simulink library "Quaternion"  (R2018b)
settings: Solver=VariableStepAuto  StartTime=0.0  StopTime=10.0  RelTol=1e-3
undefined symbols (not defined in the file): Newton, Raphson
libraries: $bdroot x8, AP_Math x3
settings Model: Creator=JCZou  LastModifiedBy=zouji
settings CodeAppCC: StateflowObjectComments=on

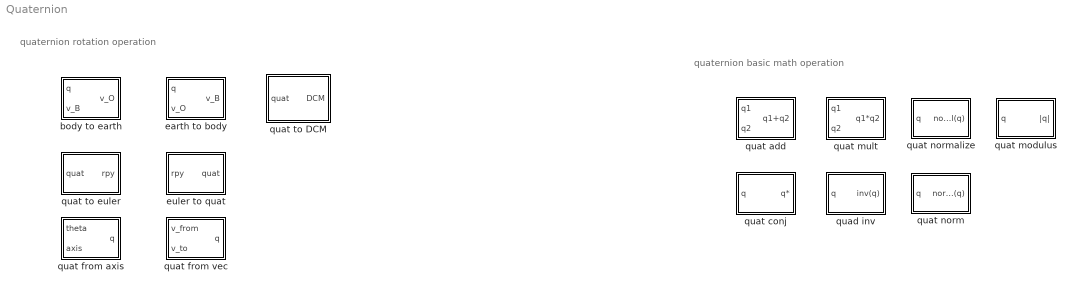
== system Quaternion ==
  note: quaternion rotation operation
  note: quaternion basic math operation
  body to earth : Subsystem
  earth to body : Subsystem
  euler to quat : Subsystem
  quad inv : Subsystem
  quat add : Subsystem
  quat conj : Subsystem
  quat from axis : Subsystem
  quat from vec : Subsystem
  quat modulus : Subsystem
  quat mult : Subsystem
  quat norm : Subsystem
  quat normalize : Subsystem
  quat to DCM : Subsystem
  quat to euler : Subsystem

== system Quaternion/body to earth ==
  q : Inport  Unit=1
  v_B : Inport  Port=2
  Mux : Mux  Inputs=3
  Subsystem : Subsystem
  Subsystem1 : Subsystem
  Subsystem2 : Subsystem
  quat normalize : $bdroot/quat normalize  SystemSampleTime=-1
  v_O : Outport
  wires:
  v_B/1 -> Subsystem/2(vec), Subsystem2/2(vec), Subsystem1/2(vec)
  quat normalize/1 -> Subsystem/1(q), Subsystem2/1(q), Subsystem1/1(q)
  Mux/1 -> v_O/1
  Subsystem1/1(V2) -> Mux/2
  Subsystem/1(V1) -> Mux/1
  Subsystem2/1(V3) -> Mux/3
  q/1 -> quat normalize/1

== system Quaternion/earth to body ==
  q : Inport  Unit=1
  v_O : Inport  Port=2
  Mux : Mux  Inputs=3
  Subsystem : Subsystem
  Subsystem1 : Subsystem
  Subsystem2 : Subsystem
  quat normalize : $bdroot/quat normalize  SystemSampleTime=-1
  v_B : Outport
  wires:
  v_O/1 -> Subsystem/2(vec), Subsystem2/2(vec), Subsystem1/2(vec)
  Subsystem1/1(V2) -> Mux/2
  Mux/1 -> v_B/1
  Subsystem/1(V1) -> Mux/1
  quat normalize/1 -> Subsystem2/1(q1), Subsystem1/1(q1), Subsystem/1(q1)
  q/1 -> quat normalize/1
  Subsystem2/1(V3) -> Mux/3

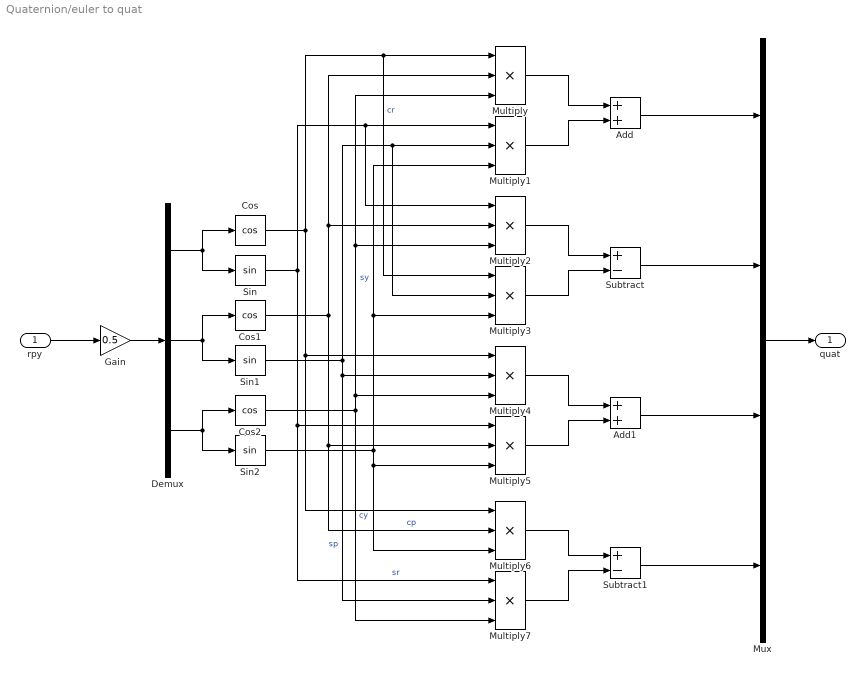
== system Quaternion/euler to quat ==
  rpy : Inport
  Add : Sum  OutDataTypeStr=Inherit: Same as first input
  Add1 : Sum  OutDataTypeStr=Inherit: Same as first input
  Cos : Trigonometry  Operator=cos
  Cos1 : Trigonometry  Operator=cos
  Cos2 : Trigonometry  Operator=cos
  Demux : Demux  Outputs=3
  Gain : Gain  Gain=0.5  OutDataTypeStr=Inherit: Same as input
  Multiply{,1..7} (8 alike) : Product  Inputs=3  OutDataTypeStr=Inherit: Same as first input
  Mux : Mux
  Sin : Trigonometry
  Sin1 : Trigonometry
  Sin2 : Trigonometry
  Subtract : Sum  Inputs=+-  OutDataTypeStr=Inherit: Same as first input
  Subtract1 : Sum  Inputs=+-  OutDataTypeStr=Inherit: Same as first input
  quat : Outport
  wires:
  rpy/1 -> Gain/1
  Gain/1 -> Demux/1
  Demux/1 -> Sin/1, Cos/1
  Demux/2 -> Cos1/1, Sin1/1
  Demux/3 -> Cos2/1, Sin2/1
  Cos/1 -> Multiply4/1, Multiply6/1, Multiply3/1, Multiply/1  "cr"
  Sin/1 -> Multiply5/1, Multiply7/1, Multiply2/1, Multiply1/1  "sr"
  Cos1/1 -> Multiply5/2, Multiply6/2, Multiply/2, Multiply2/2  "cp"
  Sin1/1 -> Multiply4/2, Multiply7/2, Multiply3/2, Multiply1/2  "sp"
  Cos2/1 -> Multiply7/3, Multiply4/3, Multiply/3, Multiply2/3  "cy"
  Sin2/1 -> Multiply5/3, Multiply6/3, Multiply1/3, Multiply3/3  "sy"
  Multiply/1 -> Add/1
  Multiply1/1 -> Add/2
  Multiply2/1 -> Subtract/1
  Multiply3/1 -> Subtract/2
  Multiply4/1 -> Add1/1
  Multiply5/1 -> Add1/2
  Multiply6/1 -> Subtract1/1
  Multiply7/1 -> Subtract1/2
  Mux/1 -> quat/1
  Add/1 -> Mux/1
  Subtract/1 -> Mux/2
  Add1/1 -> Mux/3
  Subtract1/1 -> Mux/4

== system Quaternion/quad inv ==
  q : Inport
  Divide : Product  Inputs=*/
  quat conj : $bdroot/quat conj  SystemSampleTime=-1
  quat norm : $bdroot/quat norm  SystemSampleTime=-1
  inv(q) : Outport
  wires:
  q/1 -> quat conj/1, quat norm/1
  quat conj/1 -> Divide/1
  quat norm/1 -> Divide/2
  Divide/1 -> inv(q)/1

== system Quaternion/quat add ==
  q1 : Inport
  q2 : Inport  Port=2
  Add : Sum  OutDataTypeStr=Inherit: Same as first input
  q1+q2 : Outport
  wires:
  Add/1 -> q1+q2/1
  q1/1 -> Add/1
  q2/1 -> Add/2

== system Quaternion/quat conj ==
  q : Inport
  Demux : Demux
  Gain : Gain  Gain=-1  OutDataTypeStr=Inherit: Same as input
  Gain1 : Gain  Gain=-1  OutDataTypeStr=Inherit: Same as input
  Gain2 : Gain  Gain=-1  OutDataTypeStr=Inherit: Same as input
  Mux : Mux
  q* : Outport
  wires:
  q/1 -> Demux/1
  Demux/2 -> Gain/1
  Demux/1 -> Mux/1
  Demux/3 -> Gain1/1
  Demux/4 -> Gain2/1
  Mux/1 -> q*/1
  Gain/1 -> Mux/2
  Gain1/1 -> Mux/3
  Gain2/1 -> Mux/4

== system Quaternion/quat from axis ==
  theta : Inport
  axis : Inport  Port=2
  Cos : Trigonometry  Operator=cos
  Demux : Demux  Outputs=3
  Gain : Gain  Gain=0.5  OutDataTypeStr=Inherit: Same as input
  Multiply : Product  OutDataTypeStr=Inherit: Same as first input
  Multiply1 : Product  OutDataTypeStr=Inherit: Same as first input
  Multiply2 : Product  OutDataTypeStr=Inherit: Same as first input
  Mux : Mux
  Sin : Trigonometry
  quat normalize : $bdroot/quat normalize  SystemSampleTime=-1
  q : Outport
  wires:
  theta/1 -> Gain/1
  Gain/1 -> Cos/1, Sin/1
  Mux/1 -> quat normalize/1
  Cos/1 -> Mux/1
  axis/1 -> Demux/1
  Sin/1 -> Multiply2/1, Multiply1/1, Multiply/1
  Demux/1 -> Multiply/2
  Multiply/1 -> Mux/2
  Multiply1/1 -> Mux/3
  Multiply2/1 -> Mux/4
  Demux/2 -> Multiply1/2
  Demux/3 -> Multiply2/2
  quat normalize/1 -> q/1

== system Quaternion/quat from vec ==
  v_from : Inport
  v_to : Inport  Port=2
  Acos : Trigonometry  Operator=acos
  Cos : Trigonometry  Operator=cos
  Demux : Demux  Outputs=3
  Dot Product : DotProduct  InputSameDT=on  OutDataTypeStr=Inherit: Inherit via internal rule
  Gain : Gain  Gain=0.5  OutDataTypeStr=Inherit: Same as input
  Multiply1 : Product
  Multiply2 : Product
  Multiply3 : Product
  Mux : Mux
  Sin : Trigonometry
  cross_product : AP_Math/cross_product  SystemSampleTime=-1
  quat normalize : $bdroot/quat normalize  SystemSampleTime=-1
  vec_normalize : AP_Math/vec_normalize  SystemSampleTime=-1
  vec_normalize1 : AP_Math/vec_normalize  SystemSampleTime=-1
  q : Outport
  wires:
  Mux/1 -> quat normalize/1
  v_from/1 -> vec_normalize/1
  v_to/1 -> vec_normalize1/1
  vec_normalize/1 -> cross_product/1, Dot Product/1  "a"
  vec_normalize1/1 -> cross_product/2, Dot Product/2  "b"
  Dot Product/1 -> Acos/1
  Acos/1 -> Gain/1  "theta"
  cross_product/1 -> Demux/1  "n"
  Gain/1 -> Cos/1, Sin/1
  Cos/1 -> Mux/1
  Sin/1 -> Multiply3/1, Multiply2/1, Multiply1/1
  Demux/1 -> Multiply1/2
  Multiply1/1 -> Mux/2
  Multiply2/1 -> Mux/3
  Multiply3/1 -> Mux/4
  Demux/2 -> Multiply2/2
  Demux/3 -> Multiply3/2
  quat normalize/1 -> q/1

== system Quaternion/quat modulus ==
  q : Inport  Unit=1
  quat norm : $bdroot/quat norm  SystemSampleTime=-1
  sqrt : Sqrt  AlgorithmType=Newton-Raphson  SaturateOnIntegerOverflow=on
  |q| : Outport  Unit=1
  wires:
  sqrt/1 -> |q|/1
  quat norm/1 -> sqrt/1
  q/1 -> quat norm/1

== system Quaternion/quat mult ==
  q1 : Inport  Unit=1
  q2 : Inport  Port=2  Unit=1
  Mux : Mux
  q(0) : Subsystem
  q(1) : Subsystem
  q(2) : Subsystem
  q(3) : Subsystem
  q1*q2 : Outport  Unit=1
  wires:
  q(0)/1(q0) -> Mux/1
  q2/1 -> q(0)/2(r), q(1)/2(r), q(3)/2(r), q(2)/2(r)
  q(3)/1(q4) -> Mux/4
  q1/1 -> q(0)/1(q), q(1)/1(q), q(3)/1(q), q(2)/1(q)
  q(2)/1(q3) -> Mux/3
  q(1)/1(q2) -> Mux/2
  Mux/1 -> q1*q2/1

== system Quaternion/quat norm ==
  q : Inport  Unit=1
  Demux : Demux
  Product{,1..3} (4 alike) : Product
  Sum : Sum  Inputs=4
  norm(q) : Outport  Unit=1
  wires:
  Demux/1 -> Product/1, Product/2
  Demux/3 -> Product2/1, Product2/2
  Product2/1 -> Sum/3
  Sum/1 -> norm(q)/1
  Product/1 -> Sum/1
  Product1/1 -> Sum/2
  Demux/4 -> Product3/1, Product3/2
  Product3/1 -> Sum/4
  Demux/2 -> Product1/1, Product1/2
  q/1 -> Demux/1

== system Quaternion/quat normalize ==
  q : Inport  Unit=1
  Demux : Demux
  Mux : Mux
  Product{,1..3} (4 alike) : Product  Inputs=*/
  quat modulus : $bdroot/quat modulus  SystemSampleTime=-1
  normal(q) : Outport  Unit=1
  wires:
  Demux/1 -> Product/1
  Demux/4 -> Product3/1
  Demux/3 -> Product2/1
  Demux/2 -> Product1/1
  q/1 -> quat modulus/1, Demux/1
  Mux/1 -> normal(q)/1
  quat modulus/1 -> Product3/2, Product2/2, Product/2, Product1/2
  Product/1 -> Mux/1
  Product1/1 -> Mux/2
  Product2/1 -> Mux/3
  Product3/1 -> Mux/4

== system Quaternion/quat to DCM ==
  quat : Inport
  Matrix Concatenate1 : Concatenate  NumInputs=3  Mode=Multidimensional array  ConcatenateDimension=2
  col 1 : Subsystem
  col 2 : Subsystem
  col 3 : Subsystem
  DCM : Outport
  wires:
  quat/1 -> col 3/1(q), col 2/1(q), col 1/1(q)
  col 1/1(c1) -> Matrix Concatenate1/1
  col 2/1(c2) -> Matrix Concatenate1/2
  col 3/1(c3) -> Matrix Concatenate1/3
  Matrix Concatenate1/1 -> DCM/1

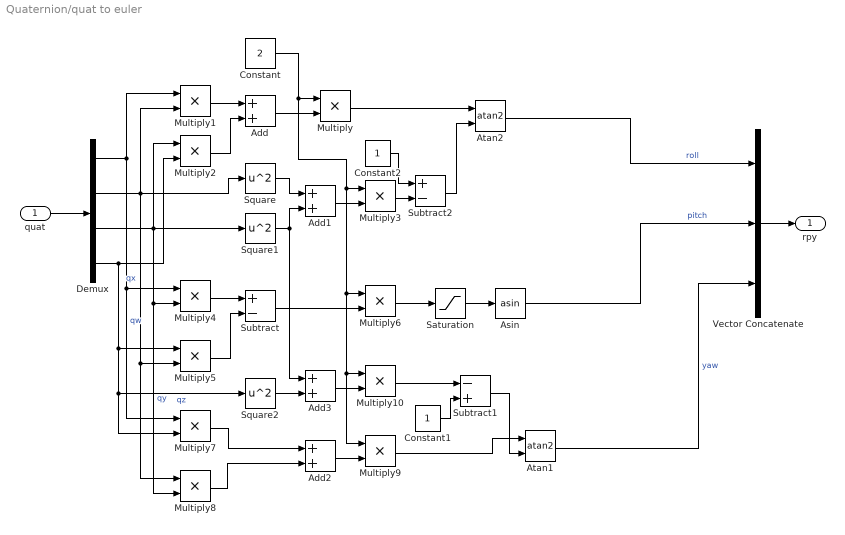
== system Quaternion/quat to euler ==
  quat : Inport
  Add{,1..3} (4 alike) : Sum
  Asin : Trigonometry  Operator=asin
  Atan1 : Trigonometry  Operator=atan2
  Atan2 : Trigonometry  Operator=atan2
  Constant : Constant  Value=2  OutDataTypeStr=single
  Constant1 : Constant  OutDataTypeStr=single
  Constant2 : Constant  OutDataTypeStr=single
  Demux : Demux
  Multiply{,1..10} (11 alike) : Product  OutDataTypeStr=Inherit: Same as first input
  Saturation : Saturate  UpperLimit=1  LowerLimit=-1
  Square : Math  Operator=square  SaturateOnIntegerOverflow=on
  Square1 : Math  Operator=square  SaturateOnIntegerOverflow=on
  Square2 : Math  Operator=square  SaturateOnIntegerOverflow=on
  Subtract : Sum  Inputs=+-
  Subtract1 : Sum  Inputs=-+
  Subtract2 : Sum  Inputs=+-
  Vector Concatenate : Concatenate  NumInputs=3
  rpy : Outport  Unit=rad
  wires:
  Vector Concatenate/1 -> rpy/1
  Square2/1 -> Add3/2
  Constant2/1 -> Subtract2/1
  Multiply3/1 -> Subtract2/2
  Demux/4 -> Square2/1, Multiply7/2, Multiply5/1, Multiply2/2  "qz"
  Multiply1/1 -> Add/1
  Add1/1 -> Multiply3/2
  Constant1/1 -> Subtract1/2
  Subtract/1 -> Multiply6/2
  Multiply10/1 -> Subtract1/1
  Square/1 -> Add1/1
  Multiply4/1 -> Subtract/1
  quat/1 -> Demux/1
  Multiply8/1 -> Add2/2
  Multiply6/1 -> Saturation/1
  Add2/1 -> Multiply9/2
  Multiply5/1 -> Subtract/2
  Multiply7/1 -> Add2/1
  Multiply/1 -> Atan2/1
  Square1/1 -> Add3/1, Add1/2
  Add3/1 -> Multiply10/2
  Multiply2/1 -> Add/2
  Demux/3 -> Multiply4/2, Multiply8/2, Square1/1, Multiply2/1  "qy"
  Demux/1 -> Multiply4/1, Multiply7/1, Multiply1/1  "qw"
  Constant/1 -> Multiply6/1, Multiply10/1, Multiply9/1, Multiply3/1, Multiply/1
  Saturation/1 -> Asin/1
  Demux/2 -> Multiply5/2, Multiply8/1, Square/1, Multiply1/2  "qx"
  Add/1 -> Multiply/2
  Multiply9/1 -> Atan1/1
  Subtract2/1 -> Atan2/2
  Subtract1/1 -> Atan1/2
  Atan2/1 -> Vector Concatenate/1  "roll"
  Asin/1 -> Vector Concatenate/2  "pitch"
  Atan1/1 -> Vector Concatenate/3  "yaw"

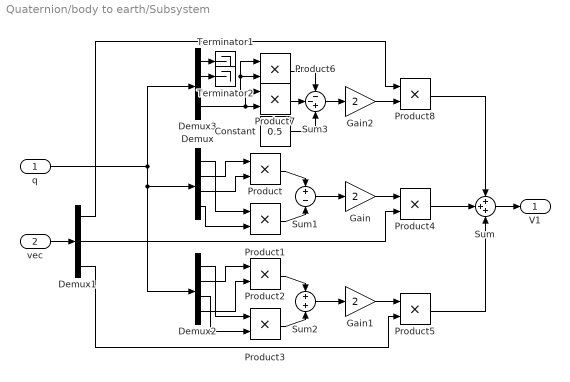
== system Quaternion/body to earth/Subsystem ==
  q : Inport
  vec : Inport  Port=2
  Constant : Constant  Value=0.5  OutDataTypeStr=single
  Demux : Demux
  Demux1 : Demux  Outputs=3
  Demux2 : Demux
  Demux3 : Demux
  Gain : Gain  Gain=2  OutDataTypeStr=Inherit: Same as input
  Gain1 : Gain  Gain=2  OutDataTypeStr=Inherit: Same as input
  Gain2 : Gain  Gain=2  OutDataTypeStr=Inherit: Same as input
  Product{,1..3,6..7} (6 alike) : Product  RndMeth=Zero
  Product4 : Product  RndMeth=Zero  OutDataTypeStr=Inherit: Same as first input
  Product5 : Product  RndMeth=Zero  OutDataTypeStr=Inherit: Same as first input
  Product8 : Product  RndMeth=Zero  OutDataTypeStr=Inherit: Same as first input
  Sum : Sum  Inputs=3  AccumDataTypeStr=single
  Sum1 : Sum  Inputs=+|-
  Sum2 : Sum  Inputs=+|+
  Sum3 : Sum  Inputs=--+
  Terminator1 : Terminator
  Terminator2 : Terminator
  V1 : Outport
  wires:
  Demux3/1 -> Terminator1/1
  Demux3/4 -> Product7/2, Product7/1
  Product8/1 -> Sum/1
  Product7/1 -> Sum3/2
  Constant/1 -> Sum3/3
  Demux1/3 -> Product5/2
  vec/1 -> Demux1/1
  Demux1/2 -> Product4/2
  Product6/1 -> Sum3/1
  Demux3/3 -> Product6/1, Product6/2
  Sum3/1 -> Gain2/1
  Gain2/1 -> Product8/2
  Gain1/1 -> Product5/1
  Gain/1 -> Product4/1
  Product4/1 -> Sum/2
  Demux1/1 -> Product8/1
  Demux3/2 -> Terminator2/1
  Sum/1 -> V1/1
  Product5/1 -> Sum/3
  Demux/4 -> Product1/2
  Sum1/1 -> Gain/1
  Product/1 -> Sum1/1
  Product1/1 -> Sum1/2
  Demux/3 -> Product/2
  Demux/1 -> Product1/1
  Demux/2 -> Product/1
  Product2/1 -> Sum2/1
  Demux2/3 -> Product3/2
  Product3/1 -> Sum2/2
  Demux2/4 -> Product2/2
  Demux2/2 -> Product2/1
  Demux2/1 -> Product3/1
  q/1 -> Demux2/1, Demux/1, Demux3/1
  Sum2/1 -> Gain1/1

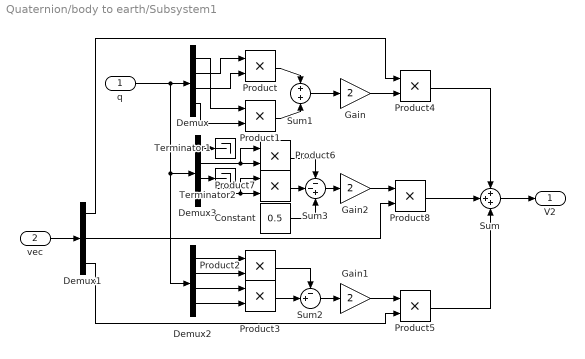
== system Quaternion/body to earth/Subsystem1 ==
  q : Inport
  vec : Inport  Port=2
  Constant : Constant  Value=0.5  OutDataTypeStr=single
  Demux : Demux
  Demux1 : Demux  Outputs=3
  Demux2 : Demux
  Demux3 : Demux
  Gain : Gain  Gain=2  OutDataTypeStr=Inherit: Same as input
  Gain1 : Gain  Gain=2  OutDataTypeStr=Inherit: Same as input
  Gain2 : Gain  Gain=2  OutDataTypeStr=Inherit: Same as input
  Product{,1..8} (9 alike) : Product  RndMeth=Zero
  Sum : Sum  Inputs=3  AccumDataTypeStr=single
  Sum1 : Sum  Inputs=+|+
  Sum2 : Sum  Inputs=-+|
  Sum3 : Sum  Inputs=--+
  Terminator1 : Terminator
  Terminator2 : Terminator
  V2 : Outport
  wires:
  Demux1/2 -> Product8/2
  Product8/1 -> Sum/2
  Demux1/1 -> Product4/1
  Product4/1 -> Sum/1
  Gain2/1 -> Product8/1
  Product5/1 -> Sum/3
  Sum/1 -> V2/1
  Demux1/3 -> Product5/2
  vec/1 -> Demux1/1
  Demux/3 -> Product/2
  Product1/1 -> Sum1/2
  Demux/1 -> Product1/1
  Demux/2 -> Product/1
  Sum1/1 -> Gain/1
  Product/1 -> Sum1/1
  Demux/4 -> Product1/2
  Gain/1 -> Product4/2
  Product7/1 -> Sum3/2
  Product6/1 -> Sum3/1
  Demux3/3 -> Terminator2/1
  Constant/1 -> Sum3/3
  Demux3/1 -> Terminator1/1
  Demux3/4 -> Product7/1, Product7/2
  Sum3/1 -> Gain2/1
  Demux3/2 -> Product6/2, Product6/1
  Product3/1 -> Sum2/2
  Product2/1 -> Sum2/1
  Demux2/4 -> Product3/2
  Demux2/1 -> Product2/1
  q/1 -> Demux/1, Demux2/1, Demux3/1
  Demux2/2 -> Product2/2
  Demux2/3 -> Product3/1
  Sum2/1 -> Gain1/1
  Gain1/1 -> Product5/1

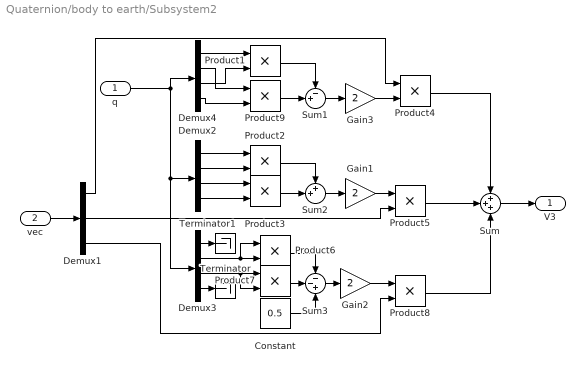
== system Quaternion/body to earth/Subsystem2 ==
  q : Inport
  vec : Inport  Port=2
  Constant : Constant  Value=0.5  OutDataTypeStr=single
  Demux1 : Demux  Outputs=3
  Demux2 : Demux
  Demux3 : Demux
  Demux4 : Demux
  Gain1 : Gain  Gain=2  OutDataTypeStr=Inherit: Same as input
  Gain2 : Gain  Gain=2  OutDataTypeStr=Inherit: Same as input
  Gain3 : Gain  Gain=2  OutDataTypeStr=Inherit: Same as input
  Product{1..9} (9 alike) : Product  RndMeth=Zero
  Sum : Sum  Inputs=3  AccumDataTypeStr=single
  Sum1 : Sum  Inputs=-+|
  Sum2 : Sum  Inputs=++|
  Sum3 : Sum  Inputs=--+
  Terminator : Terminator
  Terminator1 : Terminator
  V3 : Outport
  wires:
  vec/1 -> Demux1/1
  Demux1/1 -> Product4/1
  Product5/1 -> Sum/2
  Demux1/2 -> Product5/2
  Sum/1 -> V3/1
  Gain1/1 -> Product5/1
  Product4/1 -> Sum/1
  Gain2/1 -> Product8/1
  Gain3/1 -> Product4/2
  Product8/1 -> Sum/3
  Demux1/3 -> Product8/2
  Sum1/1 -> Gain3/1
  Demux4/1 -> Product1/1
  Demux4/4 -> Product9/2
  Demux4/2 -> Product9/1
  Product1/1 -> Sum1/1
  Product9/1 -> Sum1/2
  Demux4/3 -> Product1/2
  Sum2/1 -> Gain1/1
  Demux2/4 -> Product3/2
  Product3/1 -> Sum2/2
  Demux2/1 -> Product2/1
  Demux2/2 -> Product2/2
  Product2/1 -> Sum2/1
  Demux2/3 -> Product3/1
  Sum3/1 -> Gain2/1
  Demux3/2 -> Product6/1, Product6/2
  q/1 -> Demux4/1, Demux3/1, Demux2/1
  Constant/1 -> Sum3/3
  Product7/1 -> Sum3/2
  Product6/1 -> Sum3/1
  Demux3/3 -> Product7/2, Product7/1
  Demux3/1 -> Terminator1/1
  Demux3/4 -> Terminator/1

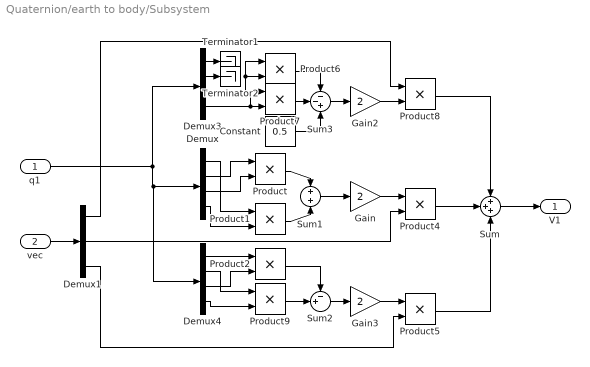
== system Quaternion/earth to body/Subsystem ==
  q1 : Inport
  vec : Inport  Port=2
  Constant : Constant  Value=0.5  OutDataTypeStr=single
  Demux : Demux
  Demux1 : Demux  Outputs=3
  Demux3 : Demux
  Demux4 : Demux
  Gain : Gain  Gain=2  OutDataTypeStr=Inherit: Same as input
  Gain2 : Gain  Gain=2  OutDataTypeStr=Inherit: Same as input
  Gain3 : Gain  Gain=2  OutDataTypeStr=Inherit: Same as input
  Product{,1..2,6..7,9} (6 alike) : Product  RndMeth=Zero
  Product4 : Product  RndMeth=Zero  OutDataTypeStr=Inherit: Same as first input
  Product5 : Product  RndMeth=Zero  OutDataTypeStr=Inherit: Same as first input
  Product8 : Product  RndMeth=Zero  OutDataTypeStr=Inherit: Same as first input
  Sum : Sum  Inputs=3  AccumDataTypeStr=single
  Sum1 : Sum  Inputs=+|+
  Sum2 : Sum  Inputs=-+|
  Sum3 : Sum  Inputs=--+
  Terminator1 : Terminator
  Terminator2 : Terminator
  V1 : Outport
  wires:
  Product6/1 -> Sum3/1
  Demux3/3 -> Product6/2, Product6/1
  Demux3/4 -> Product7/1, Product7/2
  Sum3/1 -> Gain2/1
  Constant/1 -> Sum3/3
  Product4/1 -> Sum/2
  Product5/1 -> Sum/3
  Demux1/2 -> Product4/2
  vec/1 -> Demux1/1
  Gain2/1 -> Product8/2
  Sum/1 -> V1/1
  Demux1/3 -> Product5/2
  Product7/1 -> Sum3/2
  Demux1/1 -> Product8/1
  Demux3/2 -> Terminator2/1
  Demux3/1 -> Terminator1/1
  Product8/1 -> Sum/1
  Gain/1 -> Product4/1
  Product1/1 -> Sum1/2
  Demux/1 -> Product1/1
  Demux/2 -> Product/1
  Sum1/1 -> Gain/1
  Demux/3 -> Product/2
  Product/1 -> Sum1/1
  Demux/4 -> Product1/2
  Sum2/1 -> Gain3/1
  Product9/1 -> Sum2/2
  Demux4/1 -> Product2/1
  Demux4/3 -> Product2/2
  Demux4/4 -> Product9/2
  Product2/1 -> Sum2/1
  Demux4/2 -> Product9/1
  q1/1 -> Demux3/1, Demux4/1, Demux/1
  Gain3/1 -> Product5/1

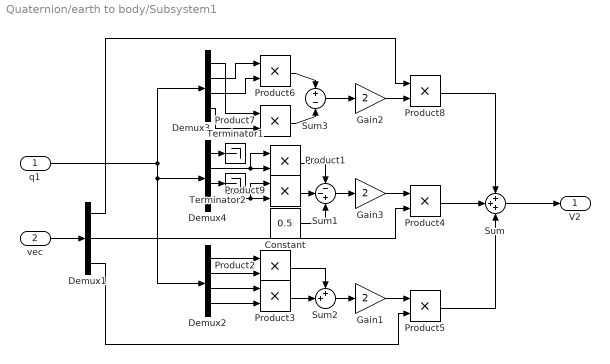
== system Quaternion/earth to body/Subsystem1 ==
  q1 : Inport
  vec : Inport  Port=2
  Constant : Constant  Value=0.5  OutDataTypeStr=single
  Demux1 : Demux  Outputs=3
  Demux2 : Demux
  Demux3 : Demux
  Demux4 : Demux
  Gain1 : Gain  Gain=2  OutDataTypeStr=Inherit: Same as input
  Gain2 : Gain  Gain=2  OutDataTypeStr=Inherit: Same as input
  Gain3 : Gain  Gain=2  OutDataTypeStr=Inherit: Same as input
  Product{1..3,6..7,9} (6 alike) : Product  RndMeth=Zero
  Product4 : Product  RndMeth=Zero  OutDataTypeStr=Inherit: Same as first input
  Product5 : Product  RndMeth=Zero  OutDataTypeStr=Inherit: Same as first input
  Product8 : Product  RndMeth=Zero  OutDataTypeStr=Inherit: Same as first input
  Sum : Sum  Inputs=3  AccumDataTypeStr=single
  Sum1 : Sum  Inputs=--+
  Sum2 : Sum  Inputs=++|
  Sum3 : Sum  Inputs=+|-
  Terminator1 : Terminator
  Terminator2 : Terminator
  V2 : Outport
  wires:
  Demux1/2 -> Product4/2
  vec/1 -> Demux1/1
  Demux1/3 -> Product5/2
  Product4/1 -> Sum/2
  Product8/1 -> Sum/1
  Sum/1 -> V2/1
  Demux1/1 -> Product8/1
  Product5/1 -> Sum/3
  Product6/1 -> Sum3/1
  Demux3/2 -> Product6/1
  Demux3/1 -> Product7/1
  Product7/1 -> Sum3/2
  Demux3/3 -> Product6/2
  Sum3/1 -> Gain2/1
  Demux3/4 -> Product7/2
  Gain2/1 -> Product8/2
  Product1/1 -> Sum1/1
  Demux4/3 -> Terminator2/1
  Sum1/1 -> Gain3/1
  Constant/1 -> Sum1/3
  Demux4/4 -> Product9/1, Product9/2
  Demux4/1 -> Terminator1/1
  Demux4/2 -> Product1/2, Product1/1
  Product9/1 -> Sum1/2
  Gain3/1 -> Product4/1
  Demux2/3 -> Product3/1
  Product2/1 -> Sum2/1
  Demux2/2 -> Product2/2
  Product3/1 -> Sum2/2
  q1/1 -> Demux2/1, Demux4/1, Demux3/1
  Demux2/4 -> Product3/2
  Sum2/1 -> Gain1/1
  Demux2/1 -> Product2/1
  Gain1/1 -> Product5/1

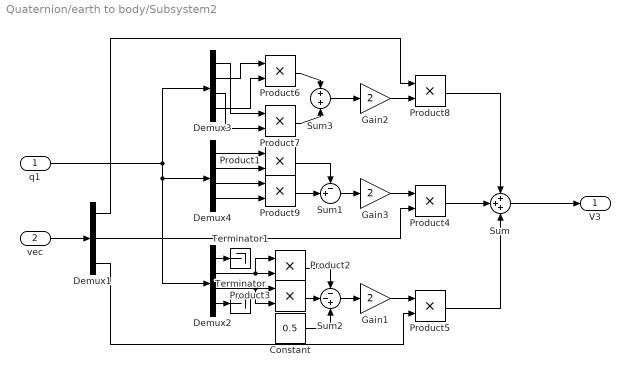
== system Quaternion/earth to body/Subsystem2 ==
  q1 : Inport
  vec : Inport  Port=2
  Constant : Constant  Value=0.5  OutDataTypeStr=single
  Demux1 : Demux  Outputs=3
  Demux2 : Demux
  Demux3 : Demux
  Demux4 : Demux
  Gain1 : Gain  Gain=2  OutDataTypeStr=Inherit: Same as input
  Gain2 : Gain  Gain=2  OutDataTypeStr=Inherit: Same as input
  Gain3 : Gain  Gain=2  OutDataTypeStr=Inherit: Same as input
  Product{1..3,6..7,9} (6 alike) : Product  RndMeth=Zero
  Product4 : Product  RndMeth=Zero  OutDataTypeStr=Inherit: Same as first input
  Product5 : Product  RndMeth=Zero  OutDataTypeStr=Inherit: Same as first input
  Product8 : Product  RndMeth=Zero  OutDataTypeStr=Inherit: Same as first input
  Sum : Sum  Inputs=3  AccumDataTypeStr=single
  Sum1 : Sum  Inputs=-+|
  Sum2 : Sum  Inputs=--+
  Sum3 : Sum  Inputs=+|+
  Terminator : Terminator
  Terminator1 : Terminator
  V3 : Outport
  wires:
  Demux1/1 -> Product8/1
  Product5/1 -> Sum/3
  Demux1/2 -> Product4/2
  vec/1 -> Demux1/1
  Demux1/3 -> Product5/2
  Product8/1 -> Sum/1
  Sum/1 -> V3/1
  Product4/1 -> Sum/2
  Product7/1 -> Sum3/2
  Demux3/3 -> Product7/2
  Sum3/1 -> Gain2/1
  Demux3/1 -> Product7/1
  Demux3/2 -> Product6/1
  Demux3/4 -> Product6/2
  Product6/1 -> Sum3/1
  Gain2/1 -> Product8/2
  Demux4/2 -> Product1/2
  Product1/1 -> Sum1/1
  Sum1/1 -> Gain3/1
  Demux4/4 -> Product9/2
  Demux4/3 -> Product9/1
  Demux4/1 -> Product1/1
  Product9/1 -> Sum1/2
  Gain3/1 -> Product4/1
  Demux2/3 -> Product3/2, Product3/1
  Demux2/1 -> Terminator1/1
  Constant/1 -> Sum2/3
  Product3/1 -> Sum2/2
  Demux2/4 -> Terminator/1
  Product2/1 -> Sum2/1
  Sum2/1 -> Gain1/1
  q1/1 -> Demux3/1, Demux2/1, Demux4/1
  Demux2/2 -> Product2/1, Product2/2
  Gain1/1 -> Product5/1

== system Quaternion/quat mult/q(0) ==
  q : Inport
  r : Inport  Port=2
  Add : Sum  Inputs=+---
  Demux : Demux
  Demux1 : Demux
  Multiply{,1..3} (4 alike) : Product  OutDataTypeStr=Inherit: Same as first input
  q0 : Outport
  wires:
  q/1 -> Demux/1
  r/1 -> Demux1/1
  Demux/1 -> Multiply/1
  Demux1/1 -> Multiply/2
  Demux/2 -> Multiply1/1
  Demux1/2 -> Multiply1/2
  Demux/3 -> Multiply2/1
  Demux1/3 -> Multiply2/2
  Demux/4 -> Multiply3/1
  Demux1/4 -> Multiply3/2
  Multiply/1 -> Add/1
  Multiply1/1 -> Add/2
  Multiply2/1 -> Add/3
  Multiply3/1 -> Add/4
  Add/1 -> q0/1

== system Quaternion/quat mult/q(1) ==
  q : Inport
  r : Inport  Port=2
  Add : Sum  Inputs=+++-
  Demux : Demux
  Demux1 : Demux
  Multiply{,1..3} (4 alike) : Product  OutDataTypeStr=Inherit: Same as first input
  q2 : Outport
  wires:
  Multiply/1 -> Add/1
  Add/1 -> q2/1
  r/1 -> Demux1/1
  q/1 -> Demux/1
  Multiply1/1 -> Add/2
  Multiply2/1 -> Add/3
  Multiply3/1 -> Add/4
  Demux/2 -> Multiply/1
  Demux1/1 -> Multiply/2
  Demux/1 -> Multiply1/1
  Demux1/2 -> Multiply1/2
  Demux/3 -> Multiply2/1
  Demux1/4 -> Multiply2/2
  Demux/4 -> Multiply3/1
  Demux1/3 -> Multiply3/2

== system Quaternion/quat mult/q(2) ==
  q : Inport
  r : Inport  Port=2
  Add : Sum  Inputs=+++-
  Demux : Demux
  Demux1 : Demux
  Multiply{,1..3} (4 alike) : Product  OutDataTypeStr=Inherit: Same as first input
  q3 : Outport
  wires:
  q/1 -> Demux/1
  Add/1 -> q3/1
  Multiply2/1 -> Add/3
  Multiply1/1 -> Add/2
  r/1 -> Demux1/1
  Multiply3/1 -> Add/4
  Multiply/1 -> Add/1
  Demux/3 -> Multiply/1
  Demux1/1 -> Multiply/2
  Demux/1 -> Multiply1/1
  Demux1/3 -> Multiply1/2
  Demux/4 -> Multiply2/1
  Demux1/2 -> Multiply2/2
  Demux/2 -> Multiply3/1
  Demux1/4 -> Multiply3/2

== system Quaternion/quat mult/q(3) ==
  q : Inport
  r : Inport  Port=2
  Add : Sum  Inputs=+++-
  Demux : Demux
  Demux1 : Demux
  Multiply{,1..3} (4 alike) : Product  OutDataTypeStr=Inherit: Same as first input
  q4 : Outport
  wires:
  r/1 -> Demux1/1
  Multiply3/1 -> Add/4
  Multiply1/1 -> Add/2
  q/1 -> Demux/1
  Multiply2/1 -> Add/3
  Add/1 -> q4/1
  Multiply/1 -> Add/1
  Demux/4 -> Multiply/1
  Demux1/1 -> Multiply/2
  Demux/1 -> Multiply1/1
  Demux1/4 -> Multiply1/2
  Demux/2 -> Multiply2/1
  Demux1/3 -> Multiply2/2
  Demux/3 -> Multiply3/1
  Demux1/2 -> Multiply3/2

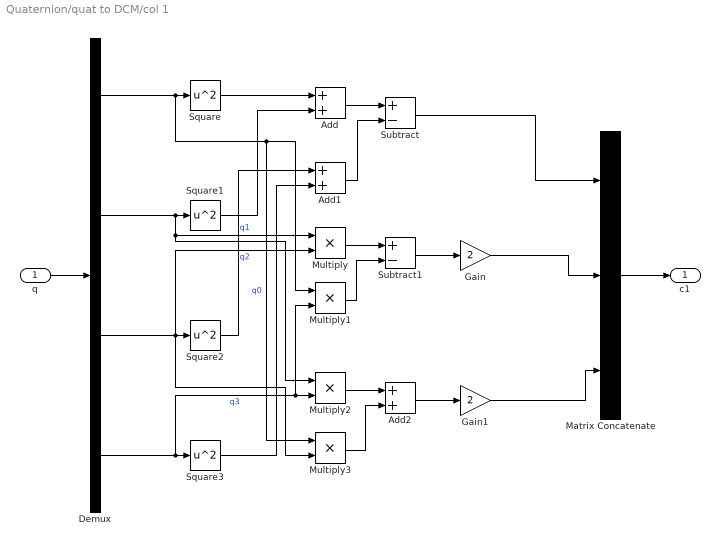
== system Quaternion/quat to DCM/col 1 ==
  q : Inport
  Add : Sum
  Add1 : Sum
  Add2 : Sum
  Demux : Demux
  Gain : Gain  Gain=2  OutDataTypeStr=Inherit: Same as input
  Gain1 : Gain  Gain=2  OutDataTypeStr=Inherit: Same as input
  Matrix Concatenate : Concatenate  NumInputs=3  ConcatenateDimension=2
  Multiply{,1..3} (4 alike) : Product  OutDataTypeStr=Inherit: Same as first input
  Square{,1..3} (4 alike) : Math  Operator=square  SaturateOnIntegerOverflow=on
  Subtract : Sum  Inputs=+-
  Subtract1 : Sum  Inputs=+-
  c1 : Outport
  wires:
  q/1 -> Demux/1
  Matrix Concatenate/1 -> c1/1
  Demux/1 -> Multiply1/1, Multiply3/1, Square/1  "q0"
  Demux/2 -> Multiply/1, Multiply2/1, Square1/1  "q1"
  Demux/3 -> Multiply/2, Square2/1, Multiply3/2  "q2"
  Demux/4 -> Multiply1/2, Multiply2/2, Square3/1  "q3"
  Square/1 -> Add/1
  Square1/1 -> Add/2
  Square2/1 -> Add1/1
  Square3/1 -> Add1/2
  Add/1 -> Subtract/1
  Add1/1 -> Subtract/2
  Subtract/1 -> Matrix Concatenate/1
  Multiply/1 -> Subtract1/1
  Multiply1/1 -> Subtract1/2
  Subtract1/1 -> Gain/1
  Gain/1 -> Matrix Concatenate/2
  Multiply2/1 -> Add2/1
  Multiply3/1 -> Add2/2
  Add2/1 -> Gain1/1
  Gain1/1 -> Matrix Concatenate/3

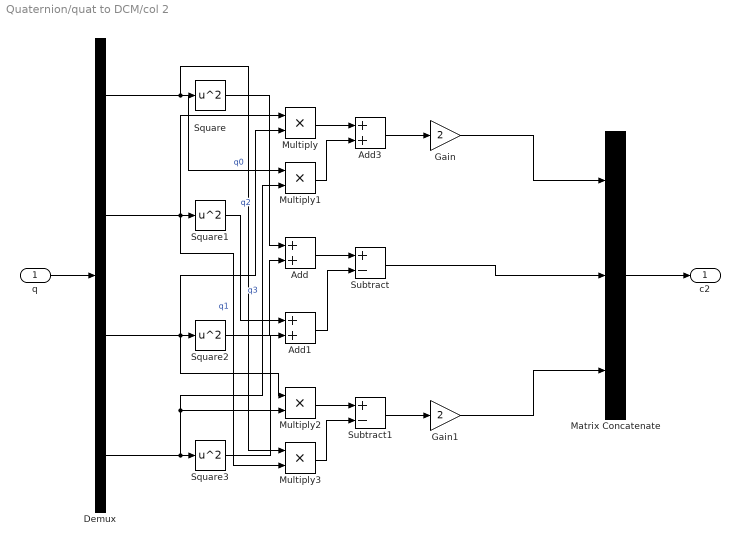
== system Quaternion/quat to DCM/col 2 ==
  q : Inport
  Add : Sum
  Add1 : Sum
  Add3 : Sum
  Demux : Demux
  Gain : Gain  Gain=2  OutDataTypeStr=Inherit: Same as input
  Gain1 : Gain  Gain=2  OutDataTypeStr=Inherit: Same as input
  Matrix Concatenate : Concatenate  NumInputs=3  ConcatenateDimension=2
  Multiply{,1..3} (4 alike) : Product  OutDataTypeStr=Inherit: Same as first input
  Square{,1..3} (4 alike) : Math  Operator=square  SaturateOnIntegerOverflow=on
  Subtract : Sum  Inputs=+-
  Subtract1 : Sum  Inputs=+-
  c2 : Outport
  wires:
  Demux/3 -> Multiply/2, Square2/1, Multiply2/1  "q2"
  Demux/1 -> Multiply1/1, Square/1, Multiply3/1  "q0"
  Matrix Concatenate/1 -> c2/1
  Demux/2 -> Multiply/1, Square1/1, Multiply3/2  "q1"
  q/1 -> Demux/1
  Demux/4 -> Multiply1/2, Multiply2/2, Square3/1  "q3"
  Add3/1 -> Gain/1
  Multiply/1 -> Add3/1
  Multiply1/1 -> Add3/2
  Gain/1 -> Matrix Concatenate/1
  Add/1 -> Subtract/1
  Add1/1 -> Subtract/2
  Square/1 -> Add/1
  Square2/1 -> Add/2
  Square1/1 -> Add1/1
  Square3/1 -> Add1/2
  Subtract/1 -> Matrix Concatenate/2
  Multiply2/1 -> Subtract1/1
  Gain1/1 -> Matrix Concatenate/3
  Multiply3/1 -> Subtract1/2
  Subtract1/1 -> Gain1/1

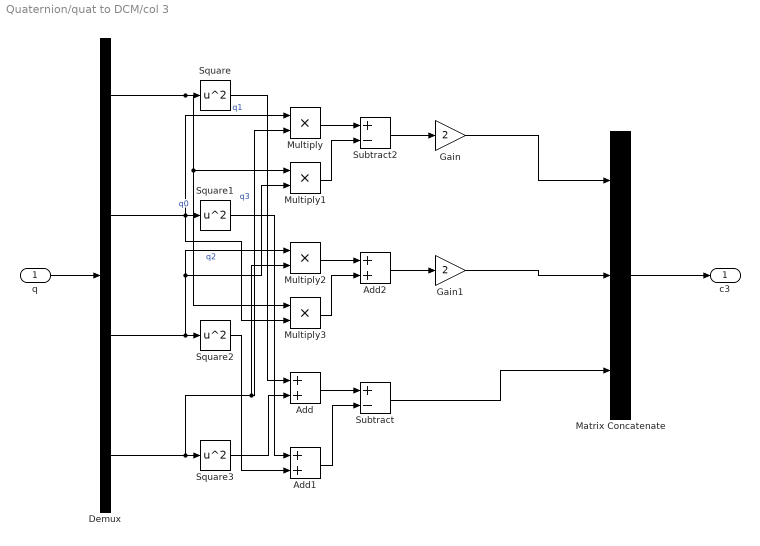
== system Quaternion/quat to DCM/col 3 ==
  q : Inport
  Add : Sum
  Add1 : Sum
  Add2 : Sum
  Demux : Demux
  Gain : Gain  Gain=2  OutDataTypeStr=Inherit: Same as input
  Gain1 : Gain  Gain=2  OutDataTypeStr=Inherit: Same as input
  Matrix Concatenate : Concatenate  NumInputs=3  ConcatenateDimension=2
  Multiply{,1..3} (4 alike) : Product  OutDataTypeStr=Inherit: Same as first input
  Square{,1..3} (4 alike) : Math  Operator=square  SaturateOnIntegerOverflow=on
  Subtract : Sum  Inputs=+-
  Subtract2 : Sum  Inputs=+-
  c3 : Outport
  wires:
  Demux/4 -> Multiply/2, Multiply2/2, Square3/1  "q3"
  Demux/3 -> Multiply1/2, Multiply2/1, Square2/1  "q2"
  Add/1 -> Subtract/1
  Multiply1/1 -> Subtract2/2
  Gain/1 -> Matrix Concatenate/1
  Add1/1 -> Subtract/2
  Add2/1 -> Gain1/1
  Multiply/1 -> Subtract2/1
  Matrix Concatenate/1 -> c3/1
  Multiply3/1 -> Add2/2
  Multiply2/1 -> Add2/1
  Subtract2/1 -> Gain/1
  Demux/1 -> Multiply1/1, Multiply3/1, Square/1  "q0"
  Demux/2 -> Multiply/1, Square1/1, Multiply3/2  "q1"
  q/1 -> Demux/1
  Square/1 -> Add/1
  Square3/1 -> Add/2
  Square1/1 -> Add1/1
  Square2/1 -> Add1/2
  Subtract/1 -> Matrix Concatenate/3
  Gain1/1 -> Matrix Concatenate/2
